simulink model "ADU_Integration_R2014a_simulation"  (R2014a)
settings: Solver=FixedStepDiscrete  StartTime=285  StopTime=300  FixedStep=0.01  RelTol=1e-3
PostLoadFcn:
  | , if any(exist('dsrtsu_mdlpostloadfcn', 'file') == [2, 3, 6]), try dsrtsu_mdlpostloadfcn('Execute', bdroot); catch fprintf('Error in PostLoadFcn (dsrtsu_mdlpostloadfcn) for model "%s":\n %s\n', bdroot, lasterr); end, end,
InitFcn:
  | load 'data/chi2_dat';
  | load 'data/Line_struct';
  | load 'data/innerLNM_1';
  | load 'data/middleLNM_2';
  | load 'data/outerLNM_1';
  | load 'data/landmarks_patac_schimmel_ccw';
  | load 'data/patac_navi_array';
  | load 'data/sensor';
  | load 'data/map_struct';
  | addpath map_src
  | Integration_Parameter;
  | load 'TestData_001';
values from neighbouring files (symbols this model uses):
  TestData_001 =     [TestData_001.mat]
undefined symbols (not defined in the file or in its folder): chi2_dat, innerLNM_1, landmarks_patac_schimmel_ccw, middleLNM_2, outerLNM_1, patac_navi_array
libraries: simulink x36, rtican x1
(part 2 of 22)

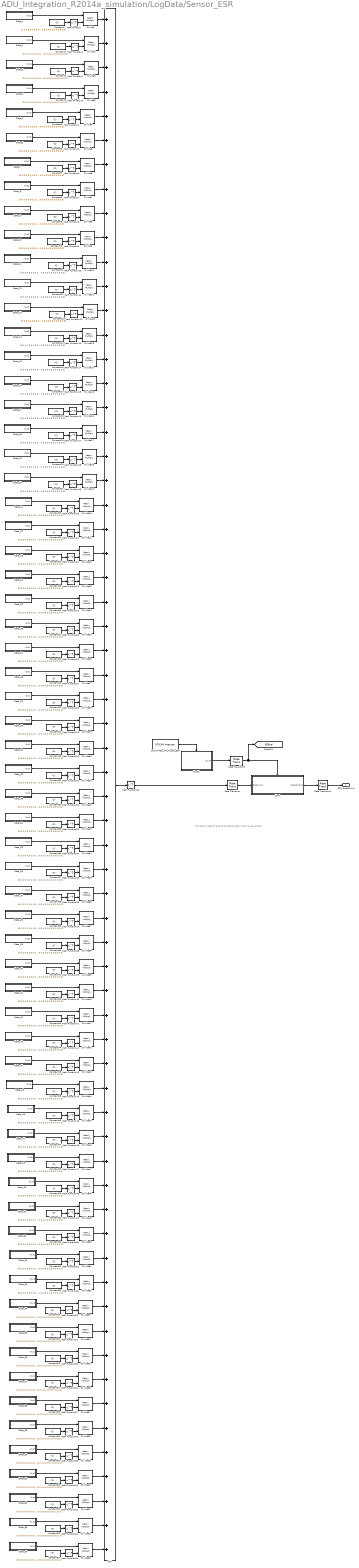
== system ADU_Integration_R2014a_simulation/LogData/Sensor_ESR ==
  note: This part is used for ensure the sensor data is from once update
  Add : Sum  Inputs=++++++++++++++++++++++++++++++++++++++++++++++++++++++++++++++++
  CAN_TYPE1_INT_M1_C1_ESR : rtican/RTICAN Interrupt  Reserved1=[]  Reserved2=[]  Reserved3=[]  Reserved4=[]  BoardTypeNo=[]  BoardNo=[]  ChannelNo=[]  Parameters=[]  InterruptName=[]  BoardIntNo=[]  Sfcn_Int_Struct=[]  BoardType=[]  SintNo=[]  Int_Struct=[]  DialogFcn=[]  UnitName=[]  Revision=[]  UnitValues=[]  DSProperties=struct('RTI',struct('Version',uint32(4),'BlockType',struct('isSLSource',uint8(1),'isSLSink',uint8(0),'isHWSource',uint8(1),'isHWSink',uint8(0),'isSetup',uint8(0),'isInline',uint8(1),'isNonInline',uint8(0),'isInterrupt',uint8(1),'isChannelwise',uint8(0)),'IOBoardType','RTICAN','UnitType','HWINT','Identifier','CANINT','DialogType','ML','BlockSet','RTICAN','RelationId',struct('TH',struct('BlockId','HWINT')),'SlaveProcessor','CAN'))  RTIBlockInterface=struct('OutputPortsWidth',int32(1),'FunctionCall',uint32(0),'OutputPortsActive',1,'DialogFcn','rtican_interrupt_gui','BlockDisplay',{{['CAN RX Interrupt'],'center'}},'IconTransparency','off','ParameterTunableNames',{{}},'InitLevel',3,'BlockName',struct('Token',{{'CAN_TYPE','_INT_M','_C'}},'BlockParam',{{'BoardTypeNo','BoardNo','ChannelNo'}}),'Options',{{'SS_OPTION_FORCE_NONINLINED_FCNCALL','SS_OPTION_ASYNCHRONOUS_INTERRUPT'}})  RTIBlockParameters=struct('BoardTypeNo',{{1,'OFF',[]}},'BoardNo',{{2,'ON',[1 16]}},'ChannelNo',{{2,'ON',[1 2]}},'Parameters',{{struct('general',struct('Type','RX','NumFormat','hex','MsgIdFormat','STD','MsgId',1343,'isFromLib',0)),'OFF',[]}},'GroupId',{{struct('Group','RTICAN','No',2,'Behavior','NAMECHANGE','BlockType','SINK','NameChangeFlag',0),'OFF',[]}},'SFcnRTICANInterrupt',{{0,'OFF',[]}},'ThSrcSgnName',{{['CAN_TYPE1_M2_C2 RX Interrupt'],'OFF',[]}},'ThBlk',{{['struct(''blkh'',''ADU_Integration_Y2016_simulation/LogData/Sensor_ESR/CAN_TYPE1_INT_M1_C1_ESR'',''srcId'',''CAN6'',''srcSgnId'',''CAN6'',''intervalTmrBlockId'',[],''srcSgnName'',[''CAN_TYPE1_M2_C2 RX Interrupt''],''srcCpuId'','''',''isSrcCpu'',1,''isTargetCpu'',1,''srcOnMasterCpu'',1,''boardType'',''CAN'',''boardTypeNo'',''1'',''boardNo'',1,''intNo'',2,''subIntNo'',-1,''period'',0,''entryPoint'',''rti_CAN6'',''blockName'',''CAN_TYPE1_INT_M1_C1_ESR'',''taskNameDisplayExt'','''',''taskType'',''HWINT'',''groupId'',''CANINT1B2'',''hookFcn'',''NULL'',''isTimerTaskSrc'',0,''service'','''',''mpBlkId'','''',''taskPriorityPreConfig'',''none'',''taskPriority'',-1,''taskSortWeighting'',[],''taskSchedulingPolicy'',''FCFS'',''taskOvrPreConfig'',''none'',''taskOvrStrategy'',1,''taskOvrQueueSize'',1,''taskVisibility'',''on'',''taskGroupId'','''',''taskGroupDisplayOrder'',[],''serviceDynamicGen'',0,''disableCodeGen'',0,''boardBase'',''0'',''noBoardBase'','''')'],'OFF',[]}},'PHSBoardBaseId',{{'DS4302','OFF',[]}},'TLCFileName',{{'rtican_interrupt','OFF',[]}})  RTISFcnParameters=struct('SFcnRTICANInterrupt','struct','ThBlk','struct','PHSBoardBaseId','char','TLCFileName','char')  RTIBlockParaDefault=struct('BoardTypeNo',4302,'BoardNo',1,'ChannelNo',1,'Parameters',struct('general',struct('Type','RX','NumFormat','dec','MsgIdFormat','STD','MsgId',100,'isFromLib',1)),'GroupId',struct('Group',{{'RTICAN'}},'No',1,'Behavior',{{'NAMECHANGE'}},'BlockType',{{'SINK'}},'NameChangeFlag',0),'SFcnRTICANInterrupt',0,'ThSrcSgnName',['DS4302CAN_B1_C1 RX Interrupt'],'ThBlk',['struct(''srcSgnId'', '''')'],'PHSBoardBaseId','DS4302','TLCFileName','rtican_interrupt')
      settings: AttributesFormatString=Group Id: RTICAN2\n
  Chart : Stateflow chart  TreatAsAtomicUnit=on
      settings: PermitHierarchicalResolution=ParametersOnly
  Chart2 : Stateflow chart  TreatAsAtomicUnit=on
      settings: PermitHierarchicalResolution=ParametersOnly
  Constant1 : Constant  Value=[0 1 0 0 0 0 0 0 0 0 0 0 0 0 0 0 0 0 0 0 0 0 0 0 0 0 0 0 0 0 0 0 0 0 0 0 0 0 0 0 0 0 0 0 0 0 0 0 0 0 0 0 0 0 0 0 0 0 0 0 0 0 0 0]
  Constant10 : Constant  Value=[0 0 0 0 0 0 0 0 0 1 0 0 0 0 0 0 0 0 0 0 0 0 0 0 0 0 0 0 0 0 0 0 0 0 0 0 0 0 0 0 0 0 0 0 0 0 0 0 0 0 0 0 0 0 0 0 0 0 0 0 0 0 0 0]
  Constant11 : Constant  Value=[0 0 0 0 0 0 0 0 0 0 1 0 0 0 0 0 0 0 0 0 0 0 0 0 0 0 0 0 0 0 0 0 0 0 0 0 0 0 0 0 0 0 0 0 0 0 0 0 0 0 0 0 0 0 0 0 0 0 0 0 0 0 0 0]
  Constant12 : Constant  Value=[0 0 0 0 0 0 0 0 0 0 0 1 0 0 0 0 0 0 0 0 0 0 0 0 0 0 0 0 0 0 0 0 0 0 0 0 0 0 0 0 0 0 0 0 0 0 0 0 0 0 0 0 0 0 0 0 0 0 0 0 0 0 0 0]
  Constant13 : Constant  Value=[0 0 0 0 0 0 0 0 0 0 0 0 1 0 0 0 0 0 0 0 0 0 0 0 0 0 0 0 0 0 0 0 0 0 0 0 0 0 0 0 0 0 0 0 0 0 0 0 0 0 0 0 0 0 0 0 0 0 0 0 0 0 0 0]
  Constant14 : Constant  Value=[0 0 0 0 0 0 0 0 0 0 0 0 0 1 0 0 0 0 0 0 0 0 0 0 0 0 0 0 0 0 0 0 0 0 0 0 0 0 0 0 0 0 0 0 0 0 0 0 0 0 0 0 0 0 0 0 0 0 0 0 0 0 0 0]
  Constant15 : Constant  Value=[0 0 0 0 0 0 0 0 0 0 0 0 0 0 0 0 0 0 0 0 0 0 0 0 0 0 0 0 0 0 0 0 0 0 0 0 0 0 0 0 0 0 0 1 0 0 0 0 0 0 0 0 0 0 0 0 0 0 0 0 0 0 0 0]
  Constant16 : Constant  Value=[0 0 0 0 0 0 0 0 0 0 0 0 0 0 1 0 0 0 0 0 0 0 0 0 0 0 0 0 0 0 0 0 0 0 0 0 0 0 0 0 0 0 0 0 0 0 0 0 0 0 0 0 0 0 0 0 0 0 0 0 0 0 0 0]
  Constant17 : Constant  Value=[0 0 0 0 0 0 0 0 0 0 0 0 0 0 0 1 0 0 0 0 0 0 0 0 0 0 0 0 0 0 0 0 0 0 0 0 0 0 0 0 0 0 0 0 0 0 0 0 0 0 0 0 0 0 0 0 0 0 0 0 0 0 0 0]
  Constant18 : Constant  Value=[0 0 0 0 0 0 0 0 0 0 0 0 0 0 0 0 1 0 0 0 0 0 0 0 0 0 0 0 0 0 0 0 0 0 0 0 0 0 0 0 0 0 0 0 0 0 0 0 0 0 0 0 0 0 0 0 0 0 0 0 0 0 0 0]
  Constant19 : Constant  Value=[0 0 0 0 0 0 0 0 0 0 0 0 0 0 0 0 0 1 0 0 0 0 0 0 0 0 0 0 0 0 0 0 0 0 0 0 0 0 0 0 0 0 0 0 0 0 0 0 0 0 0 0 0 0 0 0 0 0 0 0 0 0 0 0]
  Constant2 : Constant  Value=[0 0 1 0 0 0 0 0 0 0 0 0 0 0 0 0 0 0 0 0 0 0 0 0 0 0 0 0 0 0 0 0 0 0 0 0 0 0 0 0 0 0 0 0 0 0 0 0 0 0 0 0 0 0 0 0 0 0 0 0 0 0 0 0]
  Constant20 : Constant  Value=[0 0 0 0 0 0 0 0 0 0 0 0 0 0 0 0 0 0 1 0 0 0 0 0 0 0 0 0 0 0 0 0 0 0 0 0 0 0 0 0 0 0 0 0 0 0 0 0 0 0 0 0 0 0 0 0 0 0 0 0 0 0 0 0]
  Constant21 : Constant  Value=[0 0 0 0 0 0 0 0 0 0 0 0 0 0 0 0 0 0 0 1 0 0 0 0 0 0 0 0 0 0 0 0 0 0 0 0 0 0 0 0 0 0 0 0 0 0 0 0 0 0 0 0 0 0 0 0 0 0 0 0 0 0 0 0]
  Constant22 : Constant  Value=[0 0 0 0 0 0 0 0 0 0 0 0 0 0 0 0 0 0 0 0 1 0 0 0 0 0 0 0 0 0 0 0 0 0 0 0 0 0 0 0 0 0 0 0 0 0 0 0 0 0 0 0 0 0 0 0 0 0 0 0 0 0 0 0]
  Constant23 : Constant  Value=[0 0 0 0 0 0 0 0 0 0 0 0 0 0 0 0 0 0 0 0 0 1 0 0 0 0 0 0 0 0 0 0 0 0 0 0 0 0 0 0 0 0 0 0 0 0 0 0 0 0 0 0 0 0 0 0 0 0 0 0 0 0 0 0]
  Constant24 : Constant  Value=[0 0 0 0 0 0 0 0 0 0 0 0 0 0 0 0 0 0 0 0 0 0 1 0 0 0 0 0 0 0 0 0 0 0 0 0 0 0 0 0 0 0 0 0 0 0 0 0 0 0 0 0 0 0 0 0 0 0 0 0 0 0 0 0]
  Constant25 : Constant  Value=[0 0 0 0 0 0 0 0 0 0 0 0 0 0 0 0 0 0 0 0 0 0 0 1 0 0 0 0 0 0 0 0 0 0 0 0 0 0 0 0 0 0 0 0 0 0 0 0 0 0 0 0 0 0 0 0 0 0 0 0 0 0 0 0]
  Constant26 : Constant  Value=[0 0 0 0 0 0 0 0 0 0 0 0 0 0 0 0 0 0 0 0 0 0 0 0 1 0 0 0 0 0 0 0 0 0 0 0 0 0 0 0 0 0 0 0 0 0 0 0 0 0 0 0 0 0 0 0 0 0 0 0 0 0 0 0]
  Constant27 : Constant  Value=[0 0 0 0 0 0 0 0 0 0 0 0 0 0 0 0 0 0 0 0 0 0 0 0 0 1 0 0 0 0 0 0 0 0 0 0 0 0 0 0 0 0 0 0 0 0 0 0 0 0 0 0 0 0 0 0 0 0 0 0 0 0 0 0]
  Constant28 : Constant  Value=[0 0 0 0 0 0 0 0 0 0 0 0 0 0 0 0 0 0 0 0 0 0 0 0 0 0 1 0 0 0 0 0 0 0 0 0 0 0 0 0 0 0 0 0 0 0 0 0 0 0 0 0 0 0 0 0 0 0 0 0 0 0 0 0]
  Constant29 : Constant  Value=[0 0 0 0 0 0 0 0 0 0 0 0 0 0 0 0 0 0 0 0 0 0 0 0 0 0 0 1 0 0 0 0 0 0 0 0 0 0 0 0 0 0 0 0 0 0 0 0 0 0 0 0 0 0 0 0 0 0 0 0 0 0 0 0]
  Constant3 : Constant  Value=[0 0 0 1 0 0 0 0 0 0 0 0 0 0 0 0 0 0 0 0 0 0 0 0 0 0 0 0 0 0 0 0 0 0 0 0 0 0 0 0 0 0 0 0 0 0 0 0 0 0 0 0 0 0 0 0 0 0 0 0 0 0 0 0]
  Constant30 : Constant  Value=[0 0 0 0 0 0 0 0 0 0 0 0 0 0 0 0 0 0 0 0 0 0 0 0 0 0 0 0 1 0 0 0 0 0 0 0 0 0 0 0 0 0 0 0 0 0 0 0 0 0 0 0 0 0 0 0 0 0 0 0 0 0 0 0]
  Constant31 : Constant  Value=[0 0 0 0 0 0 0 0 0 0 0 0 0 0 0 0 0 0 0 0 0 0 0 0 0 0 0 0 0 1 0 0 0 0 0 0 0 0 0 0 0 0 0 0 0 0 0 0 0 0 0 0 0 0 0 0 0 0 0 0 0 0 0 0]
  Constant32 : Constant  Value=[0 0 0 0 0 0 0 0 0 0 0 0 0 0 0 0 0 0 0 0 0 0 0 0 0 0 0 0 0 0 1 0 0 0 0 0 0 0 0 0 0 0 0 0 0 0 0 0 0 0 0 0 0 0 0 0 0 0 0 0 0 0 0 0]
  Constant33 : Constant  Value=[0 0 0 0 0 0 0 0 0 0 0 0 0 0 0 0 0 0 0 0 0 0 0 0 0 0 0 0 0 0 0 1 0 0 0 0 0 0 0 0 0 0 0 0 0 0 0 0 0 0 0 0 0 0 0 0 0 0 0 0 0 0 0 0]
  Constant34 : Constant  Value=[0 0 0 0 0 0 0 0 0 0 0 0 0 0 0 0 0 0 0 0 0 0 0 0 0 0 0 0 0 0 0 0 1 0 0 0 0 0 0 0 0 0 0 0 0 0 0 0 0 0 0 0 0 0 0 0 0 0 0 0 0 0 0 0]
  Constant35 : Constant  Value=[0 0 0 0 0 0 0 0 0 0 0 0 0 0 0 0 0 0 0 0 0 0 0 0 0 0 0 0 0 0 0 0 0 1 0 0 0 0 0 0 0 0 0 0 0 0 0 0 0 0 0 0 0 0 0 0 0 0 0 0 0 0 0 0]
  Constant36 : Constant  Value=[0 0 0 0 0 0 0 0 0 0 0 0 0 0 0 0 0 0 0 0 0 0 0 0 0 0 0 0 0 0 0 0 0 0 1 0 0 0 0 0 0 0 0 0 0 0 0 0 0 0 0 0 0 0 0 0 0 0 0 0 0 0 0 0]
  Constant37 : Constant  Value=[0 0 0 0 0 0 0 0 0 0 0 0 0 0 0 0 0 0 0 0 0 0 0 0 0 0 0 0 0 0 0 0 0 0 0 1 0 0 0 0 0 0 0 0 0 0 0 0 0 0 0 0 0 0 0 0 0 0 0 0 0 0 0 0]
  Constant38 : Constant  Value=[0 0 0 0 0 0 0 0 0 0 0 0 0 0 0 0 0 0 0 0 0 0 0 0 0 0 0 0 0 0 0 0 0 0 0 0 1 0 0 0 0 0 0 0 0 0 0 0 0 0 0 0 0 0 0 0 0 0 0 0 0 0 0 0]
  Constant39 : Constant  Value=[0 0 0 0 0 0 0 0 0 0 0 0 0 0 0 0 0 0 0 0 0 0 0 0 0 0 0 0 0 0 0 0 0 0 0 0 0 1 0 0 0 0 0 0 0 0 0 0 0 0 0 0 0 0 0 0 0 0 0 0 0 0 0 0]
  Constant4 : Constant  Value=[1 0 0 0 0 0 0 0 0 0 0 0 0 0 0 0 0 0 0 0 0 0 0 0 0 0 0 0 0 0 0 0 0 0 0 0 0 0 0 0 0 0 0 0 0 0 0 0 0 0 0 0 0 0 0 0 0 0 0 0 0 0 0 0]
  Constant40 : Constant  Value=[0 0 0 0 0 0 0 0 0 0 0 0 0 0 0 0 0 0 0 0 0 0 0 0 0 0 0 0 0 0 0 0 0 0 0 0 0 0 1 0 0 0 0 0 0 0 0 0 0 0 0 0 0 0 0 0 0 0 0 0 0 0 0 0]
  Constant41 : Constant  Value=[0 0 0 0 0 0 0 0 0 0 0 0 0 0 0 0 0 0 0 0 0 0 0 0 0 0 0 0 0 0 0 0 0 0 0 0 0 0 0 1 0 0 0 0 0 0 0 0 0 0 0 0 0 0 0 0 0 0 0 0 0 0 0 0]
  Constant42 : Constant  Value=[0 0 0 0 0 0 0 0 0 0 0 0 0 0 0 0 0 0 0 0 0 0 0 0 0 0 0 0 0 0 0 0 0 0 0 0 0 0 0 0 1 0 0 0 0 0 0 0 0 0 0 0 0 0 0 0 0 0 0 0 0 0 0 0]
  Constant43 : Constant  Value=[0 0 0 0 0 0 0 0 0 0 0 0 0 0 0 0 0 0 0 0 0 0 0 0 0 0 0 0 0 0 0 0 0 0 0 0 0 0 0 0 0 1 0 0 0 0 0 0 0 0 0 0 0 0 0 0 0 0 0 0 0 0 0 0]
  Constant44 : Constant  Value=[0 0 0 0 0 0 0 0 0 0 0 0 0 0 0 0 0 0 0 0 0 0 0 0 0 0 0 0 0 0 0 0 0 0 0 0 0 0 0 0 0 0 1 0 0 0 0 0 0 0 0 0 0 0 0 0 0 0 0 0 0 0 0 0]
  Constant45 : Constant  Value=[0 0 0 0 0 0 0 0 0 0 0 0 0 0 0 0 0 0 0 0 0 0 0 0 0 0 0 0 0 0 0 0 0 0 0 0 0 0 0 0 0 0 0 0 1 0 0 0 0 0 0 0 0 0 0 0 0 0 0 0 0 0 0 0]
  Constant46 : Constant  Value=[0 0 0 0 0 0 0 0 0 0 0 0 0 0 0 0 0 0 0 0 0 0 0 0 0 0 0 0 0 0 0 0 0 0 0 0 0 0 0 0 0 0 0 0 0 1 0 0 0 0 0 0 0 0 0 0 0 0 0 0 0 0 0 0]
  Constant47 : Constant  Value=[0 0 0 0 0 0 0 0 0 0 0 0 0 0 0 0 0 0 0 0 0 0 0 0 0 0 0 0 0 0 0 0 0 0 0 0 0 0 0 0 0 0 0 0 0 0 1 0 0 0 0 0 0 0 0 0 0 0 0 0 0 0 0 0]
  Constant48 : Constant  Value=[0 0 0 0 0 0 0 0 0 0 0 0 0 0 0 0 0 0 0 0 0 0 0 0 0 0 0 0 0 0 0 0 0 0 0 0 0 0 0 0 0 0 0 0 0 0 0 1 0 0 0 0 0 0 0 0 0 0 0 0 0 0 0 0]
  Constant49 : Constant  Value=[0 0 0 0 0 0 0 0 0 0 0 0 0 0 0 0 0 0 0 0 0 0 0 0 0 0 0 0 0 0 0 0 0 0 0 0 0 0 0 0 0 0 0 0 0 0 0 0 1 0 0 0 0 0 0 0 0 0 0 0 0 0 0 0]
  Constant5 : Constant  Value=[0 0 0 0 1 0 0 0 0 0 0 0 0 0 0 0 0 0 0 0 0 0 0 0 0 0 0 0 0 0 0 0 0 0 0 0 0 0 0 0 0 0 0 0 0 0 0 0 0 0 0 0 0 0 0 0 0 0 0 0 0 0 0 0]
  Constant50 : Constant  Value=[0 0 0 0 0 0 0 0 0 0 0 0 0 0 0 0 0 0 0 0 0 0 0 0 0 0 0 0 0 0 0 0 0 0 0 0 0 0 0 0 0 0 0 0 0 0 0 0 0 1 0 0 0 0 0 0 0 0 0 0 0 0 0 0]
  Constant51 : Constant  Value=[0 0 0 0 0 0 0 0 0 0 0 0 0 0 0 0 0 0 0 0 0 0 0 0 0 0 0 0 0 0 0 0 0 0 0 0 0 0 0 0 0 0 0 0 0 0 0 0 0 0 1 0 0 0 0 0 0 0 0 0 0 0 0 0]
  Constant52 : Constant  Value=[0 0 0 0 0 0 0 0 0 0 0 0 0 0 0 0 0 0 0 0 0 0 0 0 0 0 0 0 0 0 0 0 0 0 0 0 0 0 0 0 0 0 0 0 0 0 0 0 0 0 0 1 0 0 0 0 0 0 0 0 0 0 0 0]
  Constant53 : Constant  Value=[0 0 0 0 0 0 0 0 0 0 0 0 0 0 0 0 0 0 0 0 0 0 0 0 0 0 0 0 0 0 0 0 0 0 0 0 0 0 0 0 0 0 0 0 0 0 0 0 0 0 0 0 1 0 0 0 0 0 0 0 0 0 0 0]
  Constant54 : Constant  Value=[0 0 0 0 0 0 0 0 0 0 0 0 0 0 0 0 0 0 0 0 0 0 0 0 0 0 0 0 0 0 0 0 0 0 0 0 0 0 0 0 0 0 0 0 0 0 0 0 0 0 0 0 0 1 0 0 0 0 0 0 0 0 0 0]
  Constant55 : Constant  Value=[0 0 0 0 0 0 0 0 0 0 0 0 0 0 0 0 0 0 0 0 0 0 0 0 0 0 0 0 0 0 0 0 0 0 0 0 0 0 0 0 0 0 0 0 0 0 0 0 0 0 0 0 0 0 1 0 0 0 0 0 0 0 0 0]
  Constant56 : Constant  Value=[0 0 0 0 0 0 0 0 0 0 0 0 0 0 0 0 0 0 0 0 0 0 0 0 0 0 0 0 0 0 0 0 0 0 0 0 0 0 0 0 0 0 0 0 0 0 0 0 0 0 0 0 0 0 0 1 0 0 0 0 0 0 0 0]
  Constant57 : Constant  Value=[0 0 0 0 0 0 0 0 0 0 0 0 0 0 0 0 0 0 0 0 0 0 0 0 0 0 0 0 0 0 0 0 0 0 0 0 0 0 0 0 0 0 0 0 0 0 0 0 0 0 0 0 0 0 0 0 1 0 0 0 0 0 0 0]
  Constant58 : Constant  Value=[0 0 0 0 0 0 0 0 0 0 0 0 0 0 0 0 0 0 0 0 0 0 0 0 0 0 0 0 0 0 0 0 0 0 0 0 0 0 0 0 0 0 0 0 0 0 0 0 0 0 0 0 0 0 0 0 0 1 0 0 0 0 0 0]
  Constant59 : Constant  Value=[0 0 0 0 0 0 0 0 0 0 0 0 0 0 0 0 0 0 0 0 0 0 0 0 0 0 0 0 0 0 0 0 0 0 0 0 0 0 0 0 0 0 0 0 0 0 0 0 0 0 0 0 0 0 0 0 0 0 1 0 0 0 0 0]
  Constant6 : Constant  Value=[0 0 0 0 0 1 0 0 0 0 0 0 0 0 0 0 0 0 0 0 0 0 0 0 0 0 0 0 0 0 0 0 0 0 0 0 0 0 0 0 0 0 0 0 0 0 0 0 0 0 0 0 0 0 0 0 0 0 0 0 0 0 0 0]
  Constant60 : Constant  Value=[0 0 0 0 0 0 0 0 0 0 0 0 0 0 0 0 0 0 0 0 0 0 0 0 0 0 0 0 0 0 0 0 0 0 0 0 0 0 0 0 0 0 0 0 0 0 0 0 0 0 0 0 0 0 0 0 0 0 0 1 0 0 0 0]
  Constant61 : Constant  Value=[0 0 0 0 0 0 0 0 0 0 0 0 0 0 0 0 0 0 0 0 0 0 0 0 0 0 0 0 0 0 0 0 0 0 0 0 0 0 0 0 0 0 0 0 0 0 0 0 0 0 0 0 0 0 0 0 0 0 0 0 1 0 0 0]
  Constant62 : Constant  Value=[0 0 0 0 0 0 0 0 0 0 0 0 0 0 0 0 0 0 0 0 0 0 0 0 0 0 0 0 0 0 0 0 0 0 0 0 0 0 0 0 0 0 0 0 0 0 0 0 0 0 0 0 0 0 0 0 0 0 0 0 0 1 0 0]
  Constant63 : Constant  Value=[0 0 0 0 0 0 0 0 0 0 0 0 0 0 0 0 0 0 0 0 0 0 0 0 0 0 0 0 0 0 0 0 0 0 0 0 0 0 0 0 0 0 0 0 0 0 0 0 0 0 0 0 0 0 0 0 0 0 0 0 0 0 1 0]
  Constant64 : Constant  Value=[0 0 0 0 0 0 0 0 0 0 0 0 0 0 0 0 0 0 0 0 0 0 0 0 0 0 0 0 0 0 0 0 0 0 0 0 0 0 0 0 0 0 0 0 0 0 0 0 0 0 0 0 0 0 0 0 0 0 0 0 0 0 0 1]
  Constant7 : Constant  Value=[0 0 0 0 0 0 1 0 0 0 0 0 0 0 0 0 0 0 0 0 0 0 0 0 0 0 0 0 0 0 0 0 0 0 0 0 0 0 0 0 0 0 0 0 0 0 0 0 0 0 0 0 0 0 0 0 0 0 0 0 0 0 0 0]
  Constant8 : Constant  Value=[0 0 0 0 0 0 0 1 0 0 0 0 0 0 0 0 0 0 0 0 0 0 0 0 0 0 0 0 0 0 0 0 0 0 0 0 0 0 0 0 0 0 0 0 0 0 0 0 0 0 0 0 0 0 0 0 0 0 0 0 0 0 0 0]
  Constant9 : Constant  Value=[0 0 0 0 0 0 0 0 1 0 0 0 0 0 0 0 0 0 0 0 0 0 0 0 0 0 0 0 0 0 0 0 0 0 0 0 0 0 0 0 0 0 0 0 0 0 0 0 0 0 0 0 0 0 0 0 0 0 0 0 0 0 0 0]
  Data_1 : Subsystem  mask{a=0}
  Data_10 : Subsystem  mask{a=9}
  Data_11 : Subsystem  mask{a=10}
  Data_12 : Subsystem  mask{a=11}
  Data_13 : Subsystem  mask{a=12}
  Data_14 : Subsystem  mask{a=13}
  Data_15 : Subsystem  mask{a=14}
  Data_16 : Subsystem  mask{a=15}
  Data_17 : Subsystem  mask{a=16}
  Data_18 : Subsystem  mask{a=17}
  Data_19 : Subsystem  mask{a=18}
  Data_2 : Subsystem  mask{a=1}
  Data_20 : Subsystem  mask{a=19}
  Data_21 : Subsystem  mask{a=20}
  Data_22 : Subsystem  mask{a=21}
  Data_23 : Subsystem  mask{a=22}
  Data_24 : Subsystem  mask{a=23}
  Data_25 : Subsystem  mask{a=24}
  Data_26 : Subsystem  mask{a=25}
  Data_27 : Subsystem  mask{a=26}
  Data_28 : Subsystem  mask{a=27}
  Data_29 : Subsystem  mask{a=28}
  Data_3 : Subsystem  mask{a=2}
  Data_30 : Subsystem  mask{a=29}
  Data_31 : Subsystem  mask{a=30}
  Data_32 : Subsystem  mask{a=31}
  Data_33 : Subsystem  mask{a=32}
  Data_34 : Subsystem  mask{a=33}
  Data_35 : Subsystem  mask{a=34}
  Data_36 : Subsystem  mask{a=35}
  Data_37 : Subsystem  mask{a=36}
  Data_38 : Subsystem  mask{a=37}
  Data_39 : Subsystem  mask{a=38}
  Data_4 : Subsystem  mask{a=3}
  Data_40 : Subsystem  mask{a=39}
  Data_41 : Subsystem  mask{a=40}
  Data_42 : Subsystem  mask{a=41}
  Data_43 : Subsystem  mask{a=42}
  Data_44 : Subsystem  mask{a=43}
  Data_45 : Subsystem  mask{a=44}
  Data_46 : Subsystem  mask{a=45}
  Data_47 : Subsystem  mask{a=46}
  Data_48 : Subsystem  mask{a=47}
  Data_49 : Subsystem  mask{a=48}
  Data_5 : Subsystem  mask{a=4}
  Data_50 : Subsystem  mask{a=49}
  Data_51 : Subsystem  mask{a=50}
  Data_52 : Subsystem  mask{a=51}
  Data_53 : Subsystem  mask{a=52}
  Data_54 : Subsystem  mask{a=53}
  Data_55 : Subsystem  mask{a=54}
  Data_56 : Subsystem  mask{a=55}
  Data_57 : Subsystem  mask{a=56}
  Data_58 : Subsystem  mask{a=57}
  Data_59 : Subsystem  mask{a=58}
  Data_6 : Subsystem  mask{a=5}
  Data_60 : Subsystem  mask{a=59}
  Data_61 : Subsystem  mask{a=60}
  Data_62 : Subsystem  mask{a=61}
  Data_63 : Subsystem  mask{a=62}
  Data_64 : Subsystem  mask{a=63}
  Data_7 : Subsystem  mask{a=6}
  Data_8 : Subsystem  mask{a=7}
  Data_9 : Subsystem  mask{a=8}
  Divide{,1..63} (64 alike) : Product  Inputs=**  Multiplication=Matrix(*)
  Math Function{,1..64} (65 alike) : Math  Operator=transpose  SaturateOnIntegerOverflow=on
  Rate Transition : RateTransition  Deterministic=off
  Rate Transition3 : RateTransition  Deterministic=off
  Rate Transition5 : RateTransition  Deterministic=off
  ESR_Data[64X4] : Outport
  tag scope: ESRcal=global
  wires:
  Constant4/1 -> Math Function/1
  Math Function/1 -> Divide/2
  Divide/1 -> Add/1
  Constant1/1 -> Math Function1/1
  Math Function1/1 -> Divide1/2
  Divide1/1 -> Add/2
  Constant2/1 -> Math Function2/1
  Math Function2/1 -> Divide2/2
  Divide2/1 -> Add/3
  Constant3/1 -> Math Function3/1
  Math Function3/1 -> Divide3/2
  Divide3/1 -> Add/4
  Constant5/1 -> Math Function4/1
  Math Function4/1 -> Divide4/2
  Divide4/1 -> Add/5
  Constant6/1 -> Math Function5/1
  Math Function5/1 -> Divide5/2
  Divide5/1 -> Add/6
  Constant7/1 -> Math Function6/1
  Math Function6/1 -> Divide6/2
  Divide6/1 -> Add/7
  Constant8/1 -> Math Function7/1
  Math Function7/1 -> Divide7/2
  Divide7/1 -> Add/8
  Constant9/1 -> Math Function8/1
  Math Function8/1 -> Divide8/2
  Divide8/1 -> Add/9
  Constant10/1 -> Math Function9/1
  Math Function9/1 -> Divide9/2
  Divide9/1 -> Add/10
  Constant11/1 -> Math Function10/1
  Math Function10/1 -> Divide10/2
  Divide10/1 -> Add/11
  Constant12/1 -> Math Function11/1
  Math Function11/1 -> Divide11/2
  Divide11/1 -> Add/12
  Constant13/1 -> Math Function12/1
  Math Function12/1 -> Divide12/2
  Divide12/1 -> Add/13
  Constant14/1 -> Math Function13/1
  Math Function13/1 -> Divide13/2
  Divide13/1 -> Add/14
  Constant16/1 -> Math Function14/1
  Math Function14/1 -> Divide14/2
  Divide14/1 -> Add/15
  Constant17/1 -> Math Function15/1
  Math Function15/1 -> Divide15/2
  Divide15/1 -> Add/16
  Constant18/1 -> Math Function16/1
  Math Function16/1 -> Divide16/2
  Divide16/1 -> Add/17
  Constant19/1 -> Math Function17/1
  Math Function17/1 -> Divide17/2
  Divide17/1 -> Add/18
  Constant20/1 -> Math Function18/1
  Math Function18/1 -> Divide18/2
  Divide18/1 -> Add/19
  Constant21/1 -> Math Function19/1
  Math Function19/1 -> Divide19/2
  Divide19/1 -> Add/20
  Constant22/1 -> Math Function20/1
  Math Function20/1 -> Divide20/2
  Divide20/1 -> Add/21
  Constant23/1 -> Math Function21/1
  Math Function21/1 -> Divide21/2
  Divide21/1 -> Add/22
  Constant24/1 -> Math Function22/1
  Math Function22/1 -> Divide22/2
  Divide22/1 -> Add/23
  Constant25/1 -> Math Function23/1
  Math Function23/1 -> Divide23/2
  Divide23/1 -> Add/24
  Constant26/1 -> Math Function24/1
  Math Function24/1 -> Divide24/2
  Divide24/1 -> Add/25
  Constant27/1 -> Math Function25/1
  Math Function25/1 -> Divide25/2
  Divide25/1 -> Add/26
  Constant28/1 -> Math Function26/1
  Math Function26/1 -> Divide26/2
  Divide26/1 -> Add/27
  Constant29/1 -> Math Function27/1
  Math Function27/1 -> Divide27/2
  Divide27/1 -> Add/28
  Constant30/1 -> Math Function28/1
  Math Function28/1 -> Divide28/2
  Divide28/1 -> Add/29
  Constant31/1 -> Math Function29/1
  Math Function29/1 -> Divide29/2
  Divide29/1 -> Add/30
  Constant32/1 -> Math Function30/1
  Math Function30/1 -> Divide30/2
  Divide30/1 -> Add/31
  Constant33/1 -> Math Function31/1
  Math Function31/1 -> Divide31/2
  Divide31/1 -> Add/32
  Constant34/1 -> Math Function32/1
  Math Function32/1 -> Divide32/2
  Divide32/1 -> Add/33
  Constant35/1 -> Math Function33/1
  Math Function33/1 -> Divide33/2
  Divide33/1 -> Add/34
  Constant36/1 -> Math Function34/1
  Math Function34/1 -> Divide34/2
  Divide34/1 -> Add/35
  Constant37/1 -> Math Function35/1
  Math Function35/1 -> Divide35/2
  Divide35/1 -> Add/36
  Constant38/1 -> Math Function36/1
  Math Function36/1 -> Divide36/2
  Divide36/1 -> Add/37
  Constant39/1 -> Math Function37/1
  Math Function37/1 -> Divide37/2
  Divide37/1 -> Add/38
  Constant40/1 -> Math Function38/1
  Divide38/1 -> Add/39
  Math Function38/1 -> Divide38/2
  Math Function45/1 -> Divide45/2
  Constant49/1 -> Math Function48/1
  Constant46/1 -> Math Function45/1
  Divide49/1 -> Add/50
  Divide45/1 -> Add/46
  Math Function48/1 -> Divide48/2
  Math Function49/1 -> Divide49/2
  Constant50/1 -> Math Function49/1
  Divide48/1 -> Add/49
  Constant41/1 -> Math Function39/1
  Math Function39/1 -> Divide39/2
  Divide39/1 -> Add/40
  Math Function40/1 -> Divide40/2
  Divide40/1 -> Add/41
  Constant42/1 -> Math Function40/1
  Constant43/1 -> Math Function41/1
  Divide41/1 -> Add/42
  Math Function41/1 -> Divide41/2
  Divide42/1 -> Add/43
  Math Function42/1 -> Divide42/2
  Constant44/1 -> Math Function42/1
  Math Function43/1 -> Divide43/2
  Divide43/1 -> Add/44
  Constant15/1 -> Math Function43/1
  Divide46/1 -> Add/47
  Math Function46/1 -> Divide46/2
  Constant47/1 -> Math Function46/1
  Constant48/1 -> Math Function47/1
  Math Function47/1 -> Divide47/2
  Divide47/1 -> Add/48
  Constant45/1 -> Math Function44/1
  Math Function44/1 -> Divide44/2
  Divide44/1 -> Add/45
  Constant54/1 -> Math Function53/1
  Math Function53/1 -> Divide53/2
  Divide53/1 -> Add/54
  Math Function54/1 -> Divide54/2
  Constant55/1 -> Math Function54/1
  Divide54/1 -> Add/55
  Math Function50/1 -> Divide50/2
  Divide50/1 -> Add/51
  Constant51/1 -> Math Function50/1
  Divide51/1 -> Add/52
  Math Function51/1 -> Divide51/2
  Constant52/1 -> Math Function51/1
  Constant56/1 -> Math Function55/1
  Math Function55/1 -> Divide55/2
  Divide55/1 -> Add/56
  Divide57/1 -> Add/58
  Math Function57/1 -> Divide57/2
  Constant58/1 -> Math Function57/1
  Constant53/1 -> Math Function52/1
  Math Function52/1 -> Divide52/2
  Divide52/1 -> Add/53
  Divide59/1 -> Add/60
  Constant60/1 -> Math Function59/1
  Math Function59/1 -> Divide59/2
  Divide56/1 -> Add/57
  Math Function56/1 -> Divide56/2
  Constant57/1 -> Math Function56/1
  Divide58/1 -> Add/59
  Math Function58/1 -> Divide58/2
  Constant59/1 -> Math Function58/1
  Divide60/1 -> Add/61
  Math Function60/1 -> Divide60/2
  Constant61/1 -> Math Function60/1
  Constant63/1 -> Math Function62/1
  Math Function62/1 -> Divide62/2
  Divide62/1 -> Add/63
  Constant62/1 -> Math Function61/1
  Math Function61/1 -> Divide61/2
  Divide61/1 -> Add/62
  Math Function63/1 -> Divide63/2
  Divide63/1 -> Add/64
  Constant64/1 -> Math Function63/1
  Add/1 -> Math Function64/1
  Math Function64/1 -> Rate Transition/1
  Chart/1(DataOutput) -> Rate Transition3/1
  Rate Transition/1 -> Chart/1(DataInput)
  Chart2/1(count) -> Rate Transition5/1
  Rate Transition5/1 -> Chart/Trigger, [ESRcal]
  CAN_TYPE1_INT_M1_C1_ESR/1 -> Chart2/Trigger
  Rate Transition3/1 -> ESR_Data[64X4]/1
  Data_1/1(Out1) -> Divide/1
  Data_2/1(Out1) -> Divide1/1
  Data_3/1(Out1) -> Divide2/1
  Data_4/1(Out1) -> Divide3/1
  Data_5/1(Out1) -> Divide4/1
  Data_6/1(Out1) -> Divide5/1
  Data_7/1(Out1) -> Divide6/1
  Data_8/1(Out1) -> Divide7/1
  Data_9/1(Out1) -> Divide8/1
  Data_10/1(Out1) -> Divide9/1
  Data_11/1(Out1) -> Divide10/1
  Data_12/1(Out1) -> Divide11/1
  Data_13/1(Out1) -> Divide12/1
  Data_14/1(Out1) -> Divide13/1
  Data_15/1(Out1) -> Divide14/1
  Data_16/1(Out1) -> Divide15/1
  Data_17/1(Out1) -> Divide16/1
  Data_18/1(Out1) -> Divide17/1
  Data_19/1(Out1) -> Divide18/1
  Data_20/1(Out1) -> Divide19/1
  Data_21/1(Out1) -> Divide20/1
  Data_22/1(Out1) -> Divide21/1
  Data_23/1(Out1) -> Divide22/1
  Data_24/1(Out1) -> Divide23/1
  Data_25/1(Out1) -> Divide24/1
  Data_26/1(Out1) -> Divide25/1
  Data_27/1(Out1) -> Divide26/1
  Data_28/1(Out1) -> Divide27/1
  Data_29/1(Out1) -> Divide28/1
  Data_30/1(Out1) -> Divide29/1
  Data_31/1(Out1) -> Divide30/1
  Data_32/1(Out1) -> Divide31/1
  Data_33/1(Out1) -> Divide32/1
  Data_34/1(Out1) -> Divide33/1
  Data_35/1(Out1) -> Divide34/1
  Data_36/1(Out1) -> Divide35/1
  Data_37/1(Out1) -> Divide36/1
  Data_38/1(Out1) -> Divide37/1
  Data_39/1(Out1) -> Divide38/1
  Data_40/1(Out1) -> Divide39/1
  Data_41/1(Out1) -> Divide40/1
  Data_42/1(Out1) -> Divide41/1
  Data_43/1(Out1) -> Divide42/1
  Data_44/1(Out1) -> Divide43/1
  Data_45/1(Out1) -> Divide44/1
  Data_46/1(Out1) -> Divide45/1
  Data_47/1(Out1) -> Divide46/1
  Data_48/1(Out1) -> Divide47/1
  Data_49/1(Out1) -> Divide48/1
  Data_50/1(Out1) -> Divide49/1
  Data_51/1(Out1) -> Divide50/1
  Data_52/1(Out1) -> Divide51/1
  Data_53/1(Out1) -> Divide52/1
  Data_54/1(Out1) -> Divide53/1
  Data_55/1(Out1) -> Divide54/1
  Data_56/1(Out1) -> Divide55/1
  Data_57/1(Out1) -> Divide56/1
  Data_58/1(Out1) -> Divide57/1
  Data_59/1(Out1) -> Divide58/1
  Data_60/1(Out1) -> Divide59/1
  Data_61/1(Out1) -> Divide60/1
  Data_62/1(Out1) -> Divide61/1
  Data_63/1(Out1) -> Divide62/1
  Data_64/1(Out1) -> Divide63/1

== system ADU_Integration_R2014a_simulation/LogData/Vision_Target ==
  note: This part is used for ensure the sensor data is from once update
  1-D Lookup Table : Lookup_n-D  NumberOfTableDimensions=1  BreakpointsForDimension1=TestData_001.X.Data  Table=TestData_001.Y(662).Data  RndMeth=Simplest  InputSameDT=on
  CameraData : Subsystem
  Chart1 : Stateflow chart  TreatAsAtomicUnit=on
      settings: PermitHierarchicalResolution=ParametersOnly
  EPM_Lane_Signals : Subsystem
  Vision_Target[25x8] : Outport
  EPM_Lane : Outport  Port=2
  tag scope: CameraCal=global, CameraTime=global
  wires:
  EPM_Lane_Signals/1(EPM_Lane_Singals) -> EPM_Lane/1
  [Clock] -> Chart1/2(Time), 1-D Lookup Table/1
  Chart1/1(Time_out) -> [CameraTime]
  1-D Lookup Table/1 -> [CameraCal], Chart1/1(Trig)
  Chart1/2(DataOutput) -> Vision_Target[25x8]/1
  CameraData/1(CameraData[25X8]) -> Chart1/3(DataInput)

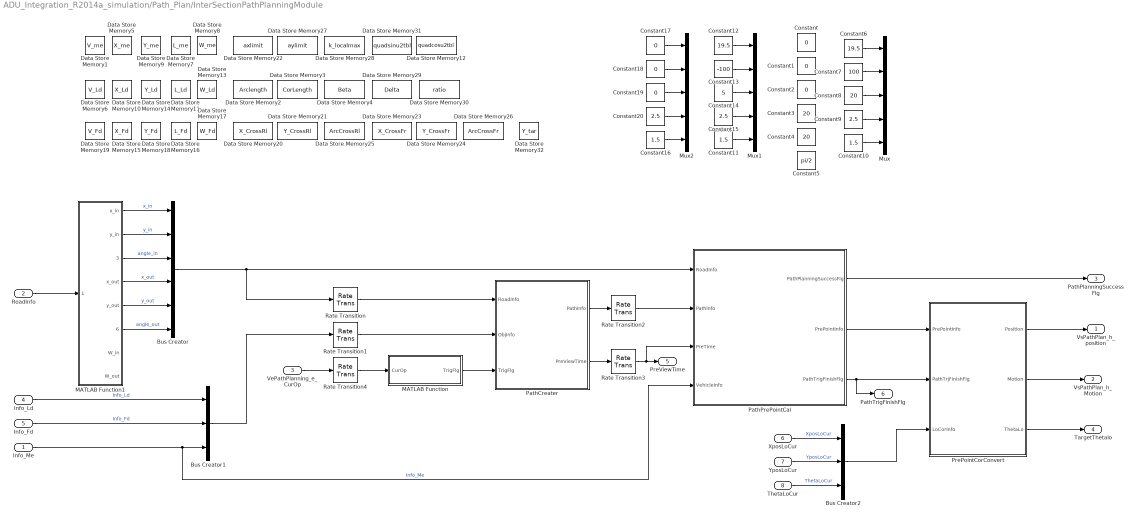
== system ADU_Integration_R2014a_simulation/Path_Plan/InterSectionPathPlanningModule ==
  Info_Me : Inport
  RoadInfo : Inport  Port=2
  VePathPlanning_e_CurOp : Inport  Port=3
  Info_Ld : Inport  Port=4
  Info_Fd : Inport  Port=5
  XposLoCur : Inport  Port=6
  YposLoCur : Inport  Port=7
  ThetaLoCur : Inport  Port=8
  Bus Creator : BusCreator  Inputs=6
  Bus Creator1 : BusCreator  Inputs=3
  Bus Creator2 : BusCreator  Inputs=3
  Constant{,1..2,17..19} (6 alike) : Constant  Value=0
  Constant10 : Constant  Value=1.5
  Constant11 : Constant  Value=1.5
  Constant12 : Constant  Value=19.5
  Constant13 : Constant  Value=-100
  Constant14 : Constant  Value=5
  Constant15 : Constant  Value=2.5
  Constant16 : Constant  Value=1.5
  Constant20 : Constant  Value=2.5
  Constant3 : Constant  Value=20
  Constant4 : Constant  Value=20
  Constant5 : Constant  Value=pi/2
  Constant6 : Constant  Value=19.5
  Constant7 : Constant  Value=100
  Constant8 : Constant  Value=20
  Constant9 : Constant  Value=2.5
  Data Store Memory1 : DataStoreMemory  DataStoreName=V_me  ReadBeforeWriteMsg=warning  WriteAfterWriteMsg=warning  WriteAfterReadMsg=warning  ShowAdditionalParam=off  OutDataTypeStr=double
  Data Store Memory10 : DataStoreMemory  DataStoreName=X_Ld  ReadBeforeWriteMsg=warning  WriteAfterWriteMsg=warning  WriteAfterReadMsg=warning  ShowAdditionalParam=off  OutDataTypeStr=double
  Data Store Memory11 : DataStoreMemory  DataStoreName=L_Ld  ReadBeforeWriteMsg=warning  WriteAfterWriteMsg=warning  WriteAfterReadMsg=warning  ShowAdditionalParam=off  OutDataTypeStr=double
  Data Store Memory12 : DataStoreMemory  DataStoreName=quadcosu2tbl  ReadBeforeWriteMsg=warning  WriteAfterWriteMsg=warning  WriteAfterReadMsg=warning  InitialValue=zeros(1,12567)  ShowAdditionalParam=off  OutDataTypeStr=double
  Data Store Memory13 : DataStoreMemory  DataStoreName=W_Ld  ReadBeforeWriteMsg=warning  WriteAfterWriteMsg=warning  WriteAfterReadMsg=warning  ShowAdditionalParam=off  OutDataTypeStr=double
  Data Store Memory14 : DataStoreMemory  DataStoreName=Y_Ld  ReadBeforeWriteMsg=warning  WriteAfterWriteMsg=warning  WriteAfterReadMsg=warning  ShowAdditionalParam=off  OutDataTypeStr=double
  Data Store Memory15 : DataStoreMemory  DataStoreName=X_Fd  ReadBeforeWriteMsg=warning  WriteAfterWriteMsg=warning  WriteAfterReadMsg=warning  ShowAdditionalParam=off  OutDataTypeStr=double
  Data Store Memory16 : DataStoreMemory  DataStoreName=L_Fd  ReadBeforeWriteMsg=warning  WriteAfterWriteMsg=warning  WriteAfterReadMsg=warning  ShowAdditionalParam=off  OutDataTypeStr=double
  Data Store Memory17 : DataStoreMemory  DataStoreName=W_Fd  ReadBeforeWriteMsg=warning  WriteAfterWriteMsg=warning  WriteAfterReadMsg=warning  ShowAdditionalParam=off  OutDataTypeStr=double
  Data Store Memory18 : DataStoreMemory  DataStoreName=Y_Fd  ReadBeforeWriteMsg=warning  WriteAfterWriteMsg=warning  WriteAfterReadMsg=warning  ShowAdditionalParam=off  OutDataTypeStr=double
  Data Store Memory19 : DataStoreMemory  DataStoreName=V_Fd  ReadBeforeWriteMsg=warning  WriteAfterWriteMsg=warning  WriteAfterReadMsg=warning  ShowAdditionalParam=off  OutDataTypeStr=double
  Data Store Memory2 : DataStoreMemory  DataStoreName=Arclength  ReadBeforeWriteMsg=warning  WriteAfterWriteMsg=warning  WriteAfterReadMsg=warning  ShowAdditionalParam=off  OutDataTypeStr=double
  Data Store Memory20 : DataStoreMemory  DataStoreName=X_CrossRl  ReadBeforeWriteMsg=warning  WriteAfterWriteMsg=warning  WriteAfterReadMsg=warning  ShowAdditionalParam=off  OutDataTypeStr=double
  Data Store Memory21 : DataStoreMemory  DataStoreName=Y_CrossRl  ReadBeforeWriteMsg=warning  WriteAfterWriteMsg=warning  WriteAfterReadMsg=warning  ShowAdditionalParam=off  OutDataTypeStr=double
  Data Store Memory22 : DataStoreMemory  DataStoreName=axlimit  ReadBeforeWriteMsg=warning  WriteAfterWriteMsg=warning  WriteAfterReadMsg=warning  ShowAdditionalParam=off  OutDataTypeStr=double
  Data Store Memory23 : DataStoreMemory  DataStoreName=X_CrossFr  ReadBeforeWriteMsg=warning  WriteAfterWriteMsg=warning  WriteAfterReadMsg=warning  ShowAdditionalParam=off  OutDataTypeStr=double
  Data Store Memory24 : DataStoreMemory  DataStoreName=Y_CrossFr  ReadBeforeWriteMsg=warning  WriteAfterWriteMsg=warning  WriteAfterReadMsg=warning  ShowAdditionalParam=off  OutDataTypeStr=double
  Data Store Memory25 : DataStoreMemory  DataStoreName=ArcCrossRl  ReadBeforeWriteMsg=warning  WriteAfterWriteMsg=warning  WriteAfterReadMsg=warning  ShowAdditionalParam=off  OutDataTypeStr=double
  Data Store Memory26 : DataStoreMemory  DataStoreName=ArcCrossFr  ReadBeforeWriteMsg=warning  WriteAfterWriteMsg=warning  WriteAfterReadMsg=warning  ShowAdditionalParam=off  OutDataTypeStr=double
  Data Store Memory27 : DataStoreMemory  DataStoreName=aylimit  ReadBeforeWriteMsg=warning  WriteAfterWriteMsg=warning  WriteAfterReadMsg=warning  ShowAdditionalParam=off  OutDataTypeStr=double
  Data Store Memory28 : DataStoreMemory  DataStoreName=k_localmax  ReadBeforeWriteMsg=warning  WriteAfterWriteMsg=warning  WriteAfterReadMsg=warning  ShowAdditionalParam=off  OutDataTypeStr=double
  Data Store Memory29 : DataStoreMemory  DataStoreName=Delta  ReadBeforeWriteMsg=warning  WriteAfterWriteMsg=warning  WriteAfterReadMsg=warning  ShowAdditionalParam=off  OutDataTypeStr=double
  Data Store Memory3 : DataStoreMemory  DataStoreName=CorLength  ReadBeforeWriteMsg=warning  WriteAfterWriteMsg=warning  WriteAfterReadMsg=warning  ShowAdditionalParam=off  OutDataTypeStr=double
  Data Store Memory30 : DataStoreMemory  DataStoreName=ratio  ReadBeforeWriteMsg=warning  WriteAfterWriteMsg=warning  WriteAfterReadMsg=warning  ShowAdditionalParam=off  OutDataTypeStr=double
  Data Store Memory31 : DataStoreMemory  DataStoreName=quadsinu2tbl  ReadBeforeWriteMsg=warning  WriteAfterWriteMsg=warning  WriteAfterReadMsg=warning  InitialValue=zeros(1,12567)  ShowAdditionalParam=off  OutDataTypeStr=double
  Data Store Memory32 : DataStoreMemory  DataStoreName=Y_tar  ReadBeforeWriteMsg=warning  WriteAfterWriteMsg=warning  WriteAfterReadMsg=warning  ShowAdditionalParam=off  OutDataTypeStr=double
  Data Store Memory4 : DataStoreMemory  DataStoreName=Beta  ReadBeforeWriteMsg=warning  WriteAfterWriteMsg=warning  WriteAfterReadMsg=warning  ShowAdditionalParam=off  OutDataTypeStr=double
  Data Store Memory5 : DataStoreMemory  DataStoreName=X_me  ReadBeforeWriteMsg=warning  WriteAfterWriteMsg=warning  WriteAfterReadMsg=warning  ShowAdditionalParam=off  OutDataTypeStr=double
  Data Store Memory6 : DataStoreMemory  DataStoreName=V_Ld  ReadBeforeWriteMsg=warning  WriteAfterWriteMsg=warning  WriteAfterReadMsg=warning  ShowAdditionalParam=off  OutDataTypeStr=double
  Data Store Memory7 : DataStoreMemory  DataStoreName=L_me  ReadBeforeWriteMsg=warning  WriteAfterWriteMsg=warning  WriteAfterReadMsg=warning  ShowAdditionalParam=off  OutDataTypeStr=double
  Data Store Memory8 : DataStoreMemory  DataStoreName=W_me  ReadBeforeWriteMsg=warning  WriteAfterWriteMsg=warning  WriteAfterReadMsg=warning  ShowAdditionalParam=off  OutDataTypeStr=double
  Data Store Memory9 : DataStoreMemory  DataStoreName=Y_me  ReadBeforeWriteMsg=warning  WriteAfterWriteMsg=warning  WriteAfterReadMsg=warning  ShowAdditionalParam=off  OutDataTypeStr=double
  MATLAB Function : MATLAB Function  TreatAsAtomicUnit=on
      settings: PermitHierarchicalResolution=ParametersOnly
  MATLAB Function1 : MATLAB Function  TreatAsAtomicUnit=on
      settings: PermitHierarchicalResolution=ParametersOnly
  Mux : Mux  Inputs=5
  Mux1 : Mux  Inputs=5
  Mux2 : Mux  Inputs=5
  PathCreater : Subsystem  TreatAsAtomicUnit=on  SystemSampleTime=0.02
  PathPrePointCal : Subsystem
  PrePointCorConvert : Subsystem  TreatAsAtomicUnit=on
  Rate Transition : RateTransition  OutPortSampleTime=0.02
  Rate Transition1 : RateTransition  OutPortSampleTime=0.02
  Rate Transition2 : RateTransition  OutPortSampleTime=0.01
  Rate Transition3 : RateTransition  OutPortSampleTime=0.01
  Rate Transition4 : RateTransition  OutPortSampleTime=0.02
  VsPathPlan_h_position : Outport
  VsPathPlan_h_Motion : Outport  Port=2
  PathPlanningSuccessFlg : Outport  Port=3
  TargetThetalo : Outport  Port=4
  PreViewTime : Outport  Port=5
  PathTrigFinishFlg : Outport  Port=6
  wires:
  Rate Transition4/1 -> MATLAB Function/1(CurOp)
  MATLAB Function/1(TrigFlg) -> PathCreater/3(TrigFlg)
  Rate Transition3/1 -> PreViewTime/1, PathPrePointCal/3(PreTime)
  VePathPlanning_e_CurOp/1 -> Rate Transition4/1
  PathPrePointCal/3(PathTrigFinishFlg) -> PrePointCorConvert/2(PathTrjFinishFlg), PathTrigFinishFlg/1
  Rate Transition2/1 -> PathPrePointCal/2(PathInfo)
  Rate Transition1/1 -> PathCreater/2(ObjInfo)
  Rate Transition/1 -> PathCreater/1(RoadInfo)
  PrePointCorConvert/3(ThetaLo) -> TargetThetalo/1
  PrePointCorConvert/2(Motion) -> VsPathPlan_h_Motion/1
  PrePointCorConvert/1(Position) -> VsPathPlan_h_position/1
  Bus Creator2/1 -> PrePointCorConvert/3(LoCorInfo)
  PathPrePointCal/2(PrePointInfo) -> PrePointCorConvert/1(PrePointInfo)
  ThetaLoCur/1 -> Bus Creator2/3  "ThetaLoCur"
  YposLoCur/1 -> Bus Creator2/2  "YposLoCur"
  XposLoCur/1 -> Bus Creator2/1  "XposLoCur"
  PathPrePointCal/1(PathPlanningSuccessFlg) -> PathPlanningSuccessFlg/1
  PathCreater/1(PathInfo) -> Rate Transition2/1
  Bus Creator1/1 -> Rate Transition1/1
  Bus Creator/1 -> PathPrePointCal/1(RoadInfo), Rate Transition/1
  MATLAB Function1/6(angle_out) -> Bus Creator/6  "angle_out"
  MATLAB Function1/5(y_out) -> Bus Creator/5  "y_out"
  MATLAB Function1/4(x_out) -> Bus Creator/4  "x_out"
  MATLAB Function1/3(angle_in) -> Bus Creator/3  "angle_in"
  MATLAB Function1/1(x_in) -> Bus Creator/1  "x_in"
  MATLAB Function1/2(y_in) -> Bus Creator/2  "y_in"
  PathCreater/2(PreViewTime) -> Rate Transition3/1
  Info_Me/1 -> PathPrePointCal/4(VehicleInfo), Bus Creator1/3  "Info_Me"
  Constant19/1 -> Mux2/3
  Constant16/1 -> Mux2/5
  Constant20/1 -> Mux2/4
  Constant18/1 -> Mux2/2
  Constant17/1 -> Mux2/1
  Info_Fd/1 -> Bus Creator1/2  "Info_Fd"
  Constant14/1 -> Mux1/3
  Constant11/1 -> Mux1/5
  Constant15/1 -> Mux1/4
  Constant13/1 -> Mux1/2
  Constant12/1 -> Mux1/1
  Info_Ld/1 -> Bus Creator1/1  "Info_Ld"
  Constant8/1 -> Mux/3
  Constant10/1 -> Mux/5
  Constant9/1 -> Mux/4
  Constant7/1 -> Mux/2
  Constant6/1 -> Mux/1
  RoadInfo/1 -> MATLAB Function1/1(RoadInfo)
